simulink model "main_sys_v1_2"  (R2015a)
settings: Solver=ode23  StartTime=0.0  StopTime=Tfin  RelTol=1e-5  AbsTol=1e-5
undefined symbols (not defined in the file): init, K, param
settings Model: Creator=jesus  LastModifiedBy=jesus
settings SolverCC: InitialStep=1e-7  SolverResetMethod=Robust
settings DataIOCC: SaveState=on

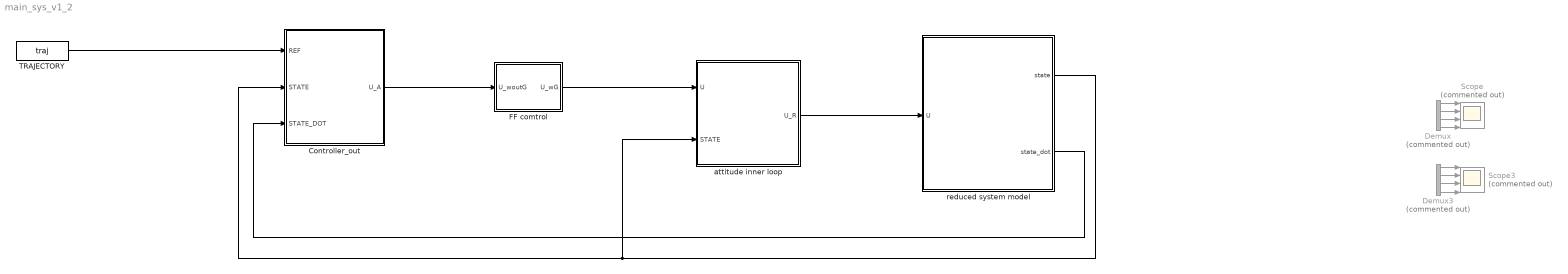
== system main_sys_v1_2 ==
  Controller_out : Subsystem
  Demux : Demux  Commented=on
  Demux3 : Demux  Commented=on
  FF comtrol : Subsystem
  Scope : Scope  Commented=on  NumInputPorts=4
      settings: YMin=-5~-5~-5~-5  YMax=5~5~5~5
  Scope3 : Scope  Commented=on  NumInputPorts=4
      settings: YMin=-5~-5~-5~-5  YMax=5~5~5~5  SaveName=ScopeData3
  TRAJECTORY : FromWorkspace  VariableName=traj  SampleTime=param.hs  Interpolate=off  OutputAfterFinalValue=Setting to zero
  attitude inner loop : Subsystem
  reduced system model : Subsystem
  wires:
  Demux/1 -> Scope/1
  Demux/2 -> Scope/2
  Demux/3 -> Scope/3
  Demux/4 -> Scope/4
  reduced system model/1(state) -> Controller_out/2(STATE), attitude inner loop/2(STATE)
  Demux3/1 -> Scope3/1
  Demux3/2 -> Scope3/2
  Demux3/3 -> Scope3/3
  Demux3/4 -> Scope3/4
  TRAJECTORY/1 -> Controller_out/1(REF)
  reduced system model/2(state_dot) -> Controller_out/3(STATE_DOT)
  attitude inner loop/1(U_R) -> reduced system model/1(U)
  Controller_out/1(U_A) -> FF comtrol/1(U_woutG)
  FF comtrol/1(U_wG) -> attitude inner loop/1(U)

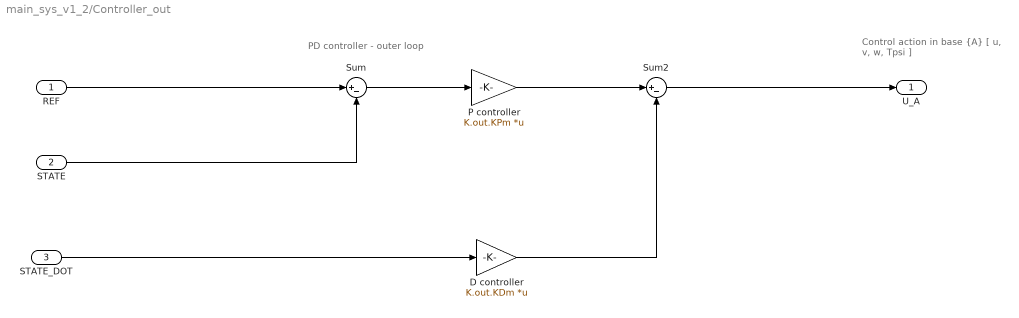
== system main_sys_v1_2/Controller_out ==
  note: Control action
      |    in base {A}
      |
      |
      |
      |
      | [ u, v, w, Tpsi ]
  note: PD controller - outer loop
  REF : Inport
  STATE : Inport  Port=2
  STATE_DOT : Inport  Port=3
  D controller : Gain  Gain=K.out.KDm  Multiplication=Matrix(K*u)
  P controller : Gain  Gain=K.out.KPm  Multiplication=Matrix(K*u)
  Sum : Sum  Inputs=|+-
  Sum2 : Sum  Inputs=|+-
  U_A : Outport
  wires:
  Sum2/1 -> U_A/1
  D controller/1 -> Sum2/2
  P controller/1 -> Sum2/1
  Sum/1 -> P controller/1
  REF/1 -> Sum/1
  STATE/1 -> Sum/2
  STATE_DOT/1 -> D controller/1

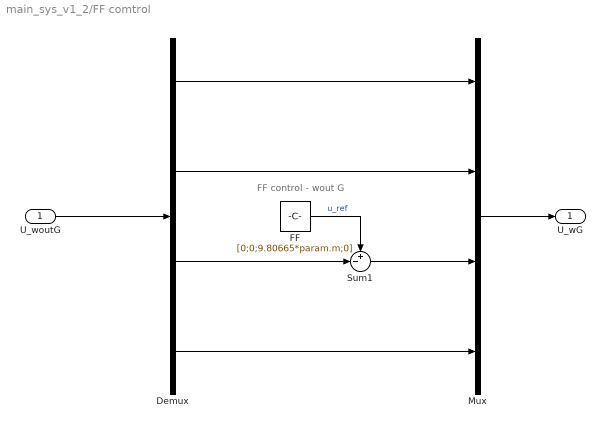
== system main_sys_v1_2/FF comtrol ==
  note: FF control - wout G
  U_woutG : Inport
  Demux : Demux
  FF : Constant  Value=[0;0;9.80665*param.m;0]
  Mux : Mux
  Sum1 : Sum  Inputs=+-|
  U_wG : Outport
  wires:
  FF/1 -> Sum1/1  "u_ref"
  Mux/1 -> U_wG/1
  U_woutG/1 -> Demux/1
  Demux/3 -> Sum1/2
  Sum1/1 -> Mux/3
  Demux/4 -> Mux/4
  Demux/2 -> Mux/2
  Demux/1 -> Mux/1

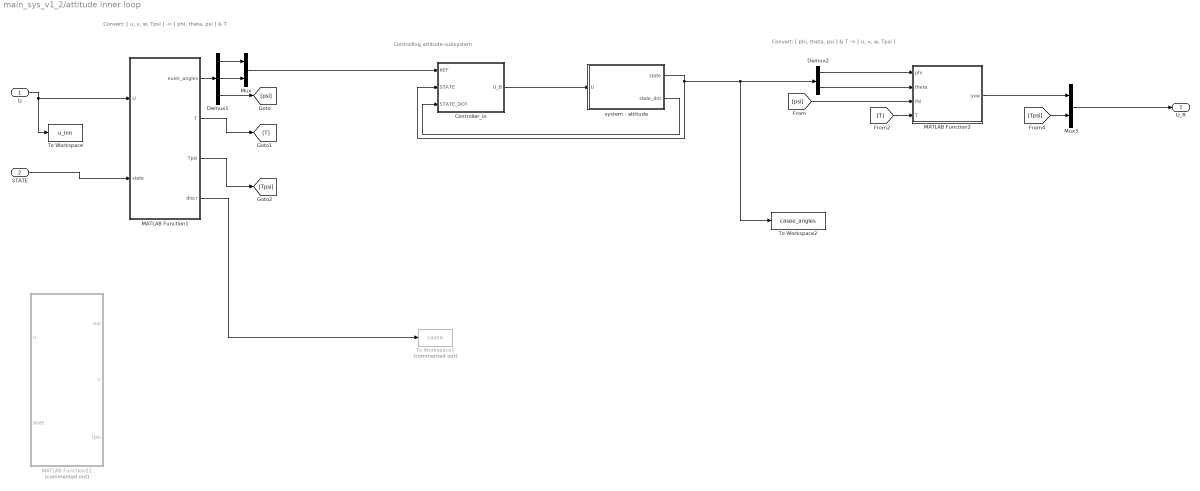
== system main_sys_v1_2/attitude inner loop ==
  note: Convert:
      |  [ phi, theta, psi ] & T -> [ u, v, w, Tpsi ]
  note: Controlling attitude subsystem
  note: Convert:
      |  [ u, v, w, Tpsi ] -> [ phi, theta, psi ] & T
  U : Inport
  STATE : Inport  Port=2
  "Controller_in " : Subsystem
  Demux1 : Demux  Outputs=3
  Demux2 : Demux  Outputs=2
  MATLAB Function1 : MATLAB Function  TreatAsAtomicUnit=on
  MATLAB Function2 : MATLAB Function  TreatAsAtomicUnit=on
  MATLAB Function22 : MATLAB Function  Commented=on  TreatAsAtomicUnit=on
  Mux : Mux  Inputs=2
  Mux3 : Mux  Inputs=2
  To Workspace : ToWorkspace  VariableName=u_inn  SaveFormat=Structure With Time  SampleTime=-1
  To Workspace1 : ToWorkspace  Commented=on  VariableName=casee  SaveFormat=Structure With Time  SampleTime=-1
  To Workspace2 : ToWorkspace  VariableName=casee_angles  SaveFormat=Structure With Time  SampleTime=-1
  system - attitude : Subsystem
  U_R : Outport
  wires:
  Demux1/1 -> Mux/1
  Demux1/2 -> Mux/2
  Demux1/3 -> [psi]
  system - attitude/1(state) -> "Controller_in "/2(STATE), To Workspace2/1, Demux2/1
  Mux/1 -> "Controller_in "/1(REF)
  system - attitude/2(state_dot) -> "Controller_in "/3(STATE_DOT)
  "Controller_in "/1(U_B) -> system - attitude/1(U)
  [T] -> MATLAB Function2/4(T)
  [Tpsi] -> Mux3/2
  MATLAB Function2/1(uvw) -> Mux3/1
  Mux3/1 -> U_R/1
  Demux2/1 -> MATLAB Function2/1(phi)
  Demux2/2 -> MATLAB Function2/2(theta)
  [psi] -> MATLAB Function2/3(Psi)
  MATLAB Function1/1(euler_angles) -> Demux1/1
  MATLAB Function1/2(T) -> [T]
  MATLAB Function1/3(Tpsi) -> [Tpsi]
  MATLAB Function1/4(discr) -> To Workspace1/1
  U/1 -> MATLAB Function1/1(U), To Workspace/1
  STATE/1 -> MATLAB Function1/2(state)

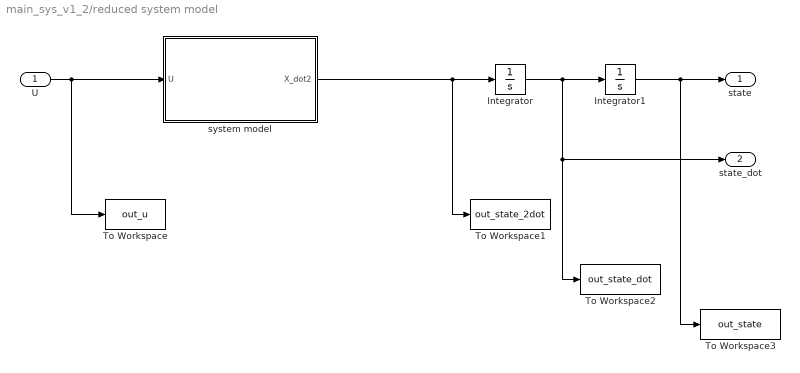
== system main_sys_v1_2/reduced system model ==
  U : Inport
  Integrator : Integrator  InitialCondition=init.out_dot
  Integrator1 : Integrator  InitialCondition=init.out
  To Workspace : ToWorkspace  VariableName=out_u  SaveFormat=Structure With Time  SampleTime=-1
  To Workspace1 : ToWorkspace  VariableName=out_state_2dot  SaveFormat=Structure With Time  SampleTime=-1
  To Workspace2 : ToWorkspace  VariableName=out_state_dot  SaveFormat=Structure With Time  SampleTime=-1
  To Workspace3 : ToWorkspace  VariableName=out_state  SaveFormat=Structure With Time  SampleTime=-1
  system model : MATLAB Function  TreatAsAtomicUnit=on
  state : Outport
  state_dot : Outport  Port=2
  wires:
  U/1 -> To Workspace/1, system model/1(U)
  Integrator/1 -> state_dot/1, To Workspace2/1, Integrator1/1
  Integrator1/1 -> To Workspace3/1, state/1
  system model/1(X_dot2) -> To Workspace1/1, Integrator/1

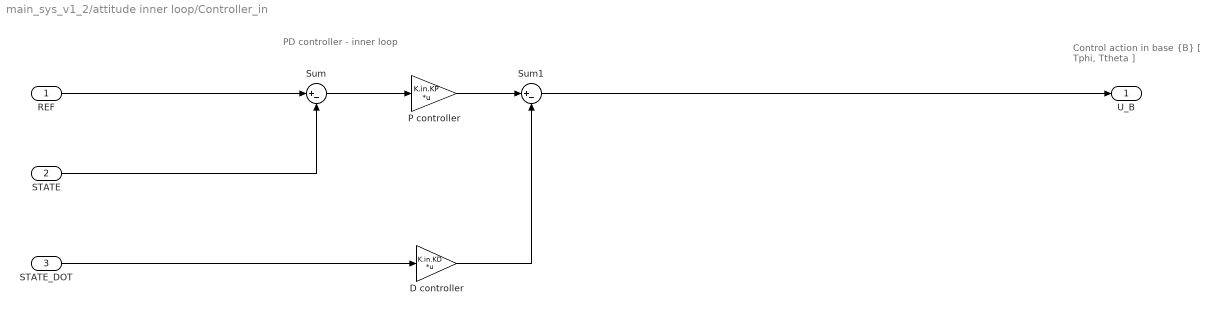
== system main_sys_v1_2/attitude inner loop/Controller_in  ==
  note: Control action
      |   in base {B}
      |
      |
      |
      | [ Tphi, Ttheta ]
  note: PD controller - inner loop
  REF : Inport
  STATE : Inport  Port=2
  STATE_DOT : Inport  Port=3
  D controller : Gain  Gain=K.in.KD  Multiplication=Matrix(K*u)
  P controller : Gain  Gain=K.in.KP  Multiplication=Matrix(K*u)
  Sum : Sum  Inputs=|+-
  Sum1 : Sum  Inputs=|+-
  U_B : Outport
  wires:
  Sum/1 -> P controller/1
  P controller/1 -> Sum1/1
  REF/1 -> Sum/1
  STATE/1 -> Sum/2
  STATE_DOT/1 -> D controller/1
  D controller/1 -> Sum1/2
  Sum1/1 -> U_B/1

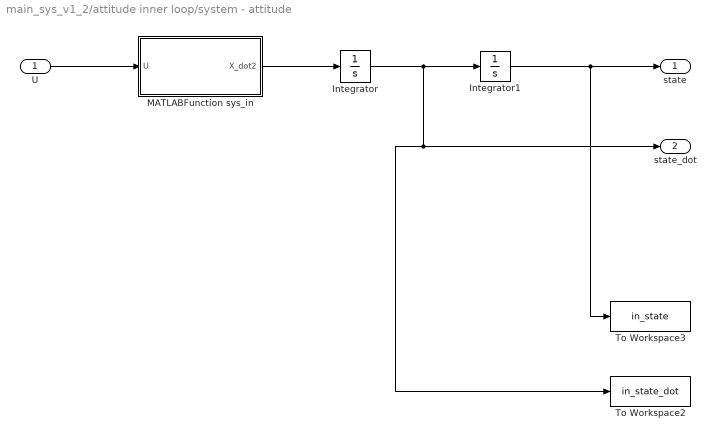
== system main_sys_v1_2/attitude inner loop/system - attitude ==
  U : Inport
  Integrator : Integrator  InitialCondition=[1e-7;1e-7]  ZeroCross=off
  Integrator1 : Integrator  InitialCondition=init.in
  MATLABFunction sys_in : MATLAB Function  TreatAsAtomicUnit=on
  To Workspace2 : ToWorkspace  VariableName=in_state_dot  SaveFormat=Structure With Time  SampleTime=-1
  To Workspace3 : ToWorkspace  VariableName=in_state  SaveFormat=Structure With Time  SampleTime=-1
  state : Outport
  state_dot : Outport  Port=2
  wires:
  U/1 -> MATLABFunction sys_in/1(U)
  Integrator/1 -> state_dot/1, To Workspace2/1, Integrator1/1
  Integrator1/1 -> To Workspace3/1, state/1
  MATLABFunction sys_in/1(X_dot2) -> Integrator/1

== matlab function main_sys_v1_2/attitude inner loop/MATLAB Function1 ==
  data: U input; euler_angles output; state input; T output; Tpsi output; discr output
function [euler_angles, T, Tpsi, discr] = fcn1(U, state)

% Mathematical derivation of formulas in XXXX

% Inputs
    u_abs = U(1);   v_abs = U(2);   w_abs = U(3);
    Tpsi = U(4);
    psi = state(4);
    
% Torque
T = sqrt( u_abs^2 + v_abs^2 + w_abs^2 );

% normalization of thrust components
u = u_abs/(T*9.80665);
v = v_abs/(T*9.80665);
w = w_abs/(T*9.80665);

% Euler angles

    % Considering w =! 0 (always true)
    %   Considering phi and theta are never 90º (iff w=!0)    

     % psi is a known value
        a = cos(psi);
        b = sin(psi);

    % compute phi & theta
    if ( u ~= 0 && v ~=0 )
        if ( a==0 )
            phi   = asinn( u/b );
            theta = atann( v/(w*b) ); 
                discr = [ 1.1; u/b; v/(w*b) ];
        elseif ( b==0 )
            phi   = asinn( -v/a );
            theta = atann( u/(w*a) );
                discr = [ 1.2; -v/a; u/(w*a) ];
        else
            aux = (u-v*w) / (b*(1+w));
            phi   = asinn( aux );
            theta = atann ( (u-b*aux) / (w*a) );
                discr = [ 1.3; aux; (u-b*aux) / (w*a) ];
        end

    elseif ( u == 0 && v == 0 )
        phi   = 0;
        theta = 0;
            discr = [ 2; 0; 0 ];

    elseif ( u == 0 && v ~= 0 )
        if ( a==0 )
            phi   = 0;
            theta = atann ( v/(b*w) );
                discr = [ 3.1; 0; v/(b*w) ];
        elseif ( b==0 )
            phi   = asinn( -v/a );
            theta = 0;
                discr = [ 3.2; -v/a; 0 ];
        else
            phi   = asinn( -a*v );
            theta = atann( b*v/w );
                discr = [ 3.3; -a*v; b*v/w ];
        end

    elseif ( u ~=0 && v == 0 )
        if ( a==0 )
            phi   = asinn( u/b );
            theta = 0;
                discr = [ 4.1; b*u; 0 ];
        elseif ( b==0 )
            phi   = 0;
            theta = atann( u/(a*w) );
                discr = [ 4.2; 0; u/(a*w) ];
        else 
            phi   = asinn( b*u );
            theta = atann( a*u/w );
                discr = [ 4.3; b*u; a*u/w ];
        end
    else
        phi = pi/3;
        theta = pi/3;
            discr = [ 5; pi/3; pi/3 ];
    end
        euler_angles = [phi; theta; psi];
end

% 
% function [ angle ] = asinn( aa )
%     angle = asin(aa);
%     % angle correction
%     if ~( -pi/2 < angle < pi/2 )
%         angle = angle - pi/2;
%     end
% end
% 
% function [ angle ] = atann( aa )
%     angle = atan(aa);
%     % angle correction
%     if ~( -pi/2 < angle < pi/2 )
%         angle = angle - pi/2;
%     end
% end

function [angle] = asinn( bb )
angle = real( asin( complex(bb) ) );
end

function [angle] = atann( bb )
angle = real( atan( complex(bb) ) );
end

== matlab function main_sys_v1_2/reduced system model/system model ==
  data: U input; X_dot2 output
function X_dot2 = syst(U)
% Simplified model of quadcopter
    % Inputs: F, Tpsi
    %   ·F: vector of forces in base{A}. projection of Thrust {B} in each
    %     direction of {A}
    %       units: [N]
    %   ·Tpsi: Torque applied around Euler's angle PSI
    %       units: [Nm]   
    %
    % Outputs: X_dot2: second derivative of the state
    %       units: ['state'/t^2]
    %
    % State: [x, y, z, psi]
    %       units: ['state']

% parameters
     m = 0.429;    g = 9.80665;   Iz = 0.00480374;

% MODEL
%   X_dot2 = (1/Mass, 1/Inertia)*(F, Tpsi) + gravity
%  

A = diag([1/m 1/m 1/m 1/Iz]);

% X_dot2 = A*U + [0; 0; -9.8; 0];

X_dot2 = zeros(4,1);
X_dot2 = A*U + [0; 0; 9.80665; 0];

== matlab function main_sys_v1_2/attitude inner loop/MATLAB Function2 ==
  data: phi input; theta input; Psi input; uvw output; T input
function uvw  = fnc2(phi, theta, Psi, T)

% call RT2uvw

% inputs
%     phi   = euler(1);
%     theta = euler(2);
%     Psi   = euler(3);
    
% rotation matrix
    R = [cos(theta)*cos(Psi),  sin(phi)*sin(theta)*cos(Psi)-cos(phi)*sin(Psi),  cos(phi)*sin(theta)*cos(Psi)+sin(phi)*sin(Psi);
         cos(theta)*sin(Psi),  sin(phi)*sin(theta)*sin(Psi)+cos(phi)*sin(Psi),  cos(phi)*sin(theta)*sin(Psi)-sin(phi)*cos(Psi);
         -sin(theta),          sin(phi)*cos(theta),                             cos(phi)*cos(theta)                           ];

    
    
%     uvw = eul2rotm( euler_angles' ) * [0;0;T];
%uvw = [];
uvw = zeros(3,1);
uvw = R*[0 0 T]';

== matlab function main_sys_v1_2/attitude inner loop/MATLAB Function22 ==
  data: U input; eul output; state input; T output; Tpsi output
function [ eul, T, Tpsi ] = U2eul( U, state )
% Mathematical derivation of formulas in XXXX
% control and coordination algorithms for autonomous multi_agent quadrotor
% systems - B.C.M. van Aert

% parameters
m = 0.429;

% Inputs
    u_abs = U(1);   v_abs = U(2);   w_abs = U(3);
    Tpsi = U(4);
    psi = state(4);
    
% Torque
T = sqrt( u_abs^2 + v_abs^2 + w_abs^2 );

% normalization of thrust components
u = u_abs/m;
v = v_abs/m;
w = w_abs/m;

% Euler angles

    % Considering w =! 0 (always true)
    %   Considering phi and theta are never 90º (iff w=!0)    

     % psi is a known value
        a = cos(psi);
        b = sin(psi);

    % compute phi & theta
    phi = asin( (v*a - u*b) / (T/m)  );
    
    theta = atan( (u*a + v*b) / (-w) );
    
    eul = [phi; theta; psi];
end

function [angle] = asinn( bb )
angle = real( asin( complex(bb) ) );
end

function [angle] = atann( bb )
angle = real( atan( complex(bb) ) );
end

== matlab function main_sys_v1_2/attitude inner loop/system - attitude/MATLABFunction sys_in ==
  data: U input; X_dot2 output
function X_dot2   = sys_in ( U )
%#codegen
% parameters
    Ix = 0.002237568100000;   
    Iy = 0.002985236000000;

X_dot2 = [ 0; 0];
X_dot2(1) = U(1) / Ix;
X_dot2(2) = U(2) / Iy;
